simulink model "MdXX_RspOutComm"  (R2018b)
settings: Solver=FixedStepDiscrete  StartTime=0.0  StopTime=10.0  FixedStep=0.01  RelTol=1e-3
undefined symbols (not defined in the file or in its folder): KeSMSuRspStatHldTm_Val
libraries: RspLib x60
(part 2 of 2)

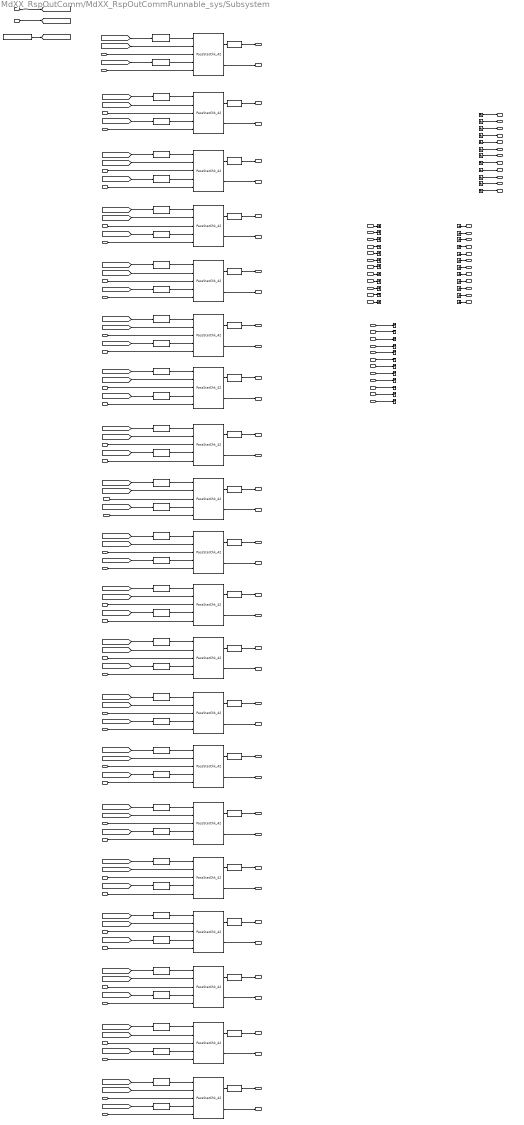
== system MdXX_RspOutComm/MdXX_RspOutCommRunnable_sys/Subsystem ==
  IsTargetPos32Bit_Val_read : Inport
  MdXX_Rsp_Md1_Rsp_read : Inport  Port=2
  MdXX_Rsp_Md10_Rsp_read : Inport  Port=3
  MdXX_Rsp_Md11_Rsp_read : Inport  Port=4
  MdXX_Rsp_Md12_Rsp_read : Inport  Port=5
  MdXX_Rsp_Md13_Rsp_read : Inport  Port=6
  MdXX_Rsp_Md14_Rsp_read : Inport  Port=7
  MdXX_Rsp_Md15_Rsp_read : Inport  Port=8
  MdXX_Rsp_Md16_Rsp_read : Inport  Port=9
  MdXX_Rsp_Md17_Rsp_read : Inport  Port=10
  MdXX_Rsp_Md18_Rsp_read : Inport  Port=11
  MdXX_Rsp_Md19_Rsp_read : Inport  Port=12
  MdXX_Rsp_Md2_Rsp_read : Inport  Port=13
  MdXX_Rsp_Md20_Rsp_read : Inport  Port=14
  MdXX_Rsp_Md21_Rsp_read : Inport  Port=15
  MdXX_Rsp_Md22_Rsp_read : Inport  Port=16
  MdXX_Rsp_Md23_Rsp_read : Inport  Port=17
  MdXX_Rsp_Md24_Rsp_read : Inport  Port=18
  MdXX_Rsp_Md25_Rsp_read : Inport  Port=19
  MdXX_Rsp_Md26_Rsp_read : Inport  Port=20
  MdXX_Rsp_Md27_Rsp_read : Inport  Port=21
  MdXX_Rsp_Md28_Rsp_read : Inport  Port=22
  MdXX_Rsp_Md29_Rsp_read : Inport  Port=23
  MdXX_Rsp_Md3_Rsp_read : Inport  Port=24
  MdXX_Rsp_Md30_Rsp_read : Inport  Port=25
  MdXX_Rsp_Md31_Rsp_read : Inport  Port=26
  MdXX_Rsp_Md32_Rsp_read : Inport  Port=27
  MdXX_Rsp_Md4_Rsp_read : Inport  Port=28
  MdXX_Rsp_Md5_Rsp_read : Inport  Port=29
  MdXX_Rsp_Md6_Rsp_read : Inport  Port=30
  MdXX_Rsp_Md7_Rsp_read : Inport  Port=31
  MdXX_Rsp_Md8_Rsp_read : Inport  Port=32
  MdXX_Rsp_Md9_Rsp_read : Inport  Port=33
  modestate32_Val_read : Inport  Port=34
  MdXX_SrcReqTp_Md1_SrcTp_read : Inport  Port=35
  MdXX_SrcReqTp_Md10_SrcTp_read : Inport  Port=36
  MdXX_SrcReqTp_Md11_SrcTp_read : Inport  Port=37
  MdXX_SrcReqTp_Md12_SrcTp_read : Inport  Port=38
  MdXX_SrcReqTp_Md13_SrcTp_read : Inport  Port=39
  MdXX_SrcReqTp_Md14_SrcTp_read : Inport  Port=40
  MdXX_SrcReqTp_Md15_SrcTp_read : Inport  Port=41
  MdXX_SrcReqTp_Md16_SrcTp_read : Inport  Port=42
  MdXX_SrcReqTp_Md17_SrcTp_read : Inport  Port=43
  MdXX_SrcReqTp_Md18_SrcTp_read : Inport  Port=44
  MdXX_SrcReqTp_Md19_SrcTp_read : Inport  Port=45
  MdXX_SrcReqTp_Md2_SrcTp_read : Inport  Port=46
  MdXX_SrcReqTp_Md20_SrcTp_read : Inport  Port=47
  MdXX_SrcReqTp_Md21_SrcTp_read : Inport  Port=48
  MdXX_SrcReqTp_Md22_SrcTp_read : Inport  Port=49
  MdXX_SrcReqTp_Md23_SrcTp_read : Inport  Port=50
  MdXX_SrcReqTp_Md24_SrcTp_read : Inport  Port=51
  MdXX_SrcReqTp_Md25_SrcTp_read : Inport  Port=52
  MdXX_SrcReqTp_Md26_SrcTp_read : Inport  Port=53
  MdXX_SrcReqTp_Md27_SrcTp_read : Inport  Port=54
  MdXX_SrcReqTp_Md28_SrcTp_read : Inport  Port=55
  MdXX_SrcReqTp_Md29_SrcTp_read : Inport  Port=56
  MdXX_SrcReqTp_Md3_SrcTp_read : Inport  Port=57
  MdXX_SrcReqTp_Md30_SrcTp_read : Inport  Port=58
  MdXX_SrcReqTp_Md31_SrcTp_read : Inport  Port=59
  MdXX_SrcReqTp_Md32_SrcTp_read : Inport  Port=60
  MdXX_SrcReqTp_Md4_SrcTp_read : Inport  Port=61
  MdXX_SrcReqTp_Md5_SrcTp_read : Inport  Port=62
  MdXX_SrcReqTp_Md6_SrcTp_read : Inport  Port=63
  MdXX_SrcReqTp_Md7_SrcTp_read : Inport  Port=64
  MdXX_SrcReqTp_Md8_SrcTp_read : Inport  Port=65
  MdXX_SrcReqTp_Md9_SrcTp_read : Inport  Port=66
  32BitSelector : RspLib/32BitSelector  BitNum=0
  32BitSelector1 : RspLib/32BitSelector  BitNum=0
  32BitSelector10 : RspLib/32BitSelector  BitNum=5
  32BitSelector11 : RspLib/32BitSelector  BitNum=5
  32BitSelector12 : RspLib/32BitSelector  BitNum=6
  32BitSelector13 : RspLib/32BitSelector  BitNum=6
  32BitSelector14 : RspLib/32BitSelector  BitNum=7
  32BitSelector15 : RspLib/32BitSelector  BitNum=7
  32BitSelector16 : RspLib/32BitSelector  BitNum=8
  32BitSelector17 : RspLib/32BitSelector  BitNum=8
  32BitSelector18 : RspLib/32BitSelector  BitNum=9
  32BitSelector19 : RspLib/32BitSelector  BitNum=9
  32BitSelector2 : RspLib/32BitSelector  BitNum=1
  32BitSelector20 : RspLib/32BitSelector  BitNum=10
  32BitSelector21 : RspLib/32BitSelector  BitNum=10
  32BitSelector22 : RspLib/32BitSelector  BitNum=11
  32BitSelector23 : RspLib/32BitSelector  BitNum=11
  32BitSelector24 : RspLib/32BitSelector  BitNum=12
  32BitSelector25 : RspLib/32BitSelector  BitNum=12
  32BitSelector26 : RspLib/32BitSelector  BitNum=13
  32BitSelector27 : RspLib/32BitSelector  BitNum=13
  32BitSelector28 : RspLib/32BitSelector  BitNum=14
  32BitSelector29 : RspLib/32BitSelector  BitNum=14
  32BitSelector3 : RspLib/32BitSelector  BitNum=1
  32BitSelector30 : RspLib/32BitSelector  BitNum=15
  32BitSelector31 : RspLib/32BitSelector  BitNum=15
  32BitSelector32 : RspLib/32BitSelector  BitNum=16
  32BitSelector33 : RspLib/32BitSelector  BitNum=16
  32BitSelector34 : RspLib/32BitSelector  BitNum=17
  32BitSelector35 : RspLib/32BitSelector  BitNum=17
  32BitSelector36 : RspLib/32BitSelector  BitNum=18
  32BitSelector37 : RspLib/32BitSelector  BitNum=18
  32BitSelector38 : RspLib/32BitSelector  BitNum=19
  32BitSelector39 : RspLib/32BitSelector  BitNum=19
  32BitSelector4 : RspLib/32BitSelector  BitNum=2
  32BitSelector5 : RspLib/32BitSelector  BitNum=2
  32BitSelector6 : RspLib/32BitSelector  BitNum=3
  32BitSelector7 : RspLib/32BitSelector  BitNum=3
  32BitSelector8 : RspLib/32BitSelector  BitNum=4
  32BitSelector9 : RspLib/32BitSelector  BitNum=4
  Data Type Conversion{1..20} (20 alike) : DataTypeConversion  OutDataTypeStr=uint8
  Ground_{1..12,14..22,24..26} (24 alike) : Ground
  Md10RspOutComm : RspLib/PassStatChk_42  SystemSampleTime=-1
  Md11RspOutComm : RspLib/PassStatChk_42  SystemSampleTime=-1
  Md12RspOutComm : RspLib/PassStatChk_42  SystemSampleTime=-1
  Md13RspOutComm : RspLib/PassStatChk_42  SystemSampleTime=-1
  Md14RspOutComm : RspLib/PassStatChk_42  SystemSampleTime=-1
  Md15RspOutComm : RspLib/PassStatChk_42  SystemSampleTime=-1
  Md16RspOutComm : RspLib/PassStatChk_42  SystemSampleTime=-1
  Md17RspOutComm : RspLib/PassStatChk_42  SystemSampleTime=-1
  Md18RspOutComm : RspLib/PassStatChk_42  SystemSampleTime=-1
  Md19RspOutComm : RspLib/PassStatChk_42  SystemSampleTime=-1
  Md1RspOutComm : RspLib/PassStatChk_42  SystemSampleTime=-1
  Md20RspOutComm : RspLib/PassStatChk_42  SystemSampleTime=-1
  Md2RspOutComm : RspLib/PassStatChk_42  SystemSampleTime=-1
  Md3RspOutComm : RspLib/PassStatChk_42  SystemSampleTime=-1
  Md4RspOutComm : RspLib/PassStatChk_42  SystemSampleTime=-1
  Md5RspOutComm : RspLib/PassStatChk_42  SystemSampleTime=-1
  Md6RspOutComm : RspLib/PassStatChk_42  SystemSampleTime=-1
  Md7RspOutComm : RspLib/PassStatChk_42  SystemSampleTime=-1
  Md8RspOutComm : RspLib/PassStatChk_42  SystemSampleTime=-1
  Md9RspOutComm : RspLib/PassStatChk_42  SystemSampleTime=-1
  PA_KeSMSuRspStatHldTm_Val : Constant  Value=KeSMSuRspStatHldTm_Val
  Terminator_{1..12,15..23,25..27} (24 alike) : Terminator
  MdXX_RspOutComm_Md1_Rsp_write : Outport
      settings: EnsureOutportIsVirtual=on
  MdXX_RspOutComm_Md10_Rsp_write : Outport  Port=2
      settings: EnsureOutportIsVirtual=on
  MdXX_RspOutComm_Md11_Rsp_write : Outport  Port=3
      settings: EnsureOutportIsVirtual=on
  MdXX_RspOutComm_Md12_Rsp_write : Outport  Port=4
      settings: EnsureOutportIsVirtual=on
  MdXX_RspOutComm_Md13_Rsp_write : Outport  Port=5
      settings: EnsureOutportIsVirtual=on
  MdXX_RspOutComm_Md14_Rsp_write : Outport  Port=6
      settings: EnsureOutportIsVirtual=on
  MdXX_RspOutComm_Md15_Rsp_write : Outport  Port=7
      settings: EnsureOutportIsVirtual=on
  MdXX_RspOutComm_Md16_Rsp_write : Outport  Port=8
      settings: EnsureOutportIsVirtual=on
  MdXX_RspOutComm_Md17_Rsp_write : Outport  Port=9
      settings: EnsureOutportIsVirtual=on
  MdXX_RspOutComm_Md18_Rsp_write : Outport  Port=10
      settings: EnsureOutportIsVirtual=on
  MdXX_RspOutComm_Md19_Rsp_write : Outport  Port=11
      settings: EnsureOutportIsVirtual=on
  MdXX_RspOutComm_Md2_Rsp_write : Outport  Port=12
      settings: EnsureOutportIsVirtual=on
  MdXX_RspOutComm_Md20_Rsp_write : Outport  Port=13
      settings: EnsureOutportIsVirtual=on
  MdXX_RspOutComm_Md21_Rsp_write : Outport  Port=14
      settings: EnsureOutportIsVirtual=on
  MdXX_RspOutComm_Md22_Rsp_write : Outport  Port=15
      settings: EnsureOutportIsVirtual=on
  MdXX_RspOutComm_Md23_Rsp_write : Outport  Port=16
      settings: EnsureOutportIsVirtual=on
  MdXX_RspOutComm_Md24_Rsp_write : Outport  Port=17
      settings: EnsureOutportIsVirtual=on
  MdXX_RspOutComm_Md25_Rsp_write : Outport  Port=18
      settings: EnsureOutportIsVirtual=on
  MdXX_RspOutComm_Md26_Rsp_write : Outport  Port=19
      settings: EnsureOutportIsVirtual=on
  MdXX_RspOutComm_Md27_Rsp_write : Outport  Port=20
      settings: EnsureOutportIsVirtual=on
  MdXX_RspOutComm_Md28_Rsp_write : Outport  Port=21
      settings: EnsureOutportIsVirtual=on
  MdXX_RspOutComm_Md29_Rsp_write : Outport  Port=22
      settings: EnsureOutportIsVirtual=on
  MdXX_RspOutComm_Md3_Rsp_write : Outport  Port=23
      settings: EnsureOutportIsVirtual=on
  MdXX_RspOutComm_Md30_Rsp_write : Outport  Port=24
      settings: EnsureOutportIsVirtual=on
  MdXX_RspOutComm_Md31_Rsp_write : Outport  Port=25
      settings: EnsureOutportIsVirtual=on
  MdXX_RspOutComm_Md32_Rsp_write : Outport  Port=26
      settings: EnsureOutportIsVirtual=on
  MdXX_RspOutComm_Md4_Rsp_write : Outport  Port=27
      settings: EnsureOutportIsVirtual=on
  MdXX_RspOutComm_Md5_Rsp_write : Outport  Port=28
      settings: EnsureOutportIsVirtual=on
  MdXX_RspOutComm_Md6_Rsp_write : Outport  Port=29
      settings: EnsureOutportIsVirtual=on
  MdXX_RspOutComm_Md7_Rsp_write : Outport  Port=30
      settings: EnsureOutportIsVirtual=on
  MdXX_RspOutComm_Md8_Rsp_write : Outport  Port=31
      settings: EnsureOutportIsVirtual=on
  MdXX_RspOutComm_Md9_Rsp_write : Outport  Port=32
      settings: EnsureOutportIsVirtual=on
  MdXX_SrcReqTpOutComm_Md1_SrcTp_write : Outport  Port=33
      settings: EnsureOutportIsVirtual=on
  MdXX_SrcReqTpOutComm_Md10_SrcTp_write : Outport  Port=34
      settings: EnsureOutportIsVirtual=on
  MdXX_SrcReqTpOutComm_Md11_SrcTp_write : Outport  Port=35
      settings: EnsureOutportIsVirtual=on
  MdXX_SrcReqTpOutComm_Md12_SrcTp_write : Outport  Port=36
      settings: EnsureOutportIsVirtual=on
  MdXX_SrcReqTpOutComm_Md13_SrcTp_write : Outport  Port=37
      settings: EnsureOutportIsVirtual=on
  MdXX_SrcReqTpOutComm_Md14_SrcTp_write : Outport  Port=38
      settings: EnsureOutportIsVirtual=on
  MdXX_SrcReqTpOutComm_Md15_SrcTp_write : Outport  Port=39
      settings: EnsureOutportIsVirtual=on
  MdXX_SrcReqTpOutComm_Md16_SrcTp_write : Outport  Port=40
      settings: EnsureOutportIsVirtual=on
  MdXX_SrcReqTpOutComm_Md17_SrcTp_write : Outport  Port=41
      settings: EnsureOutportIsVirtual=on
  MdXX_SrcReqTpOutComm_Md18_SrcTp_write : Outport  Port=42
      settings: EnsureOutportIsVirtual=on
  MdXX_SrcReqTpOutComm_Md19_SrcTp_write : Outport  Port=43
      settings: EnsureOutportIsVirtual=on
  MdXX_SrcReqTpOutComm_Md2_SrcTp_write : Outport  Port=44
      settings: EnsureOutportIsVirtual=on
  MdXX_SrcReqTpOutComm_Md20_SrcTp_write : Outport  Port=45
      settings: EnsureOutportIsVirtual=on
  MdXX_SrcReqTpOutComm_Md21_SrcTp_write : Outport  Port=46
      settings: EnsureOutportIsVirtual=on
  MdXX_SrcReqTpOutComm_Md22_SrcTp_write : Outport  Port=47
      settings: EnsureOutportIsVirtual=on
  MdXX_SrcReqTpOutComm_Md23_SrcTp_write : Outport  Port=48
      settings: EnsureOutportIsVirtual=on
  MdXX_SrcReqTpOutComm_Md24_SrcTp_write : Outport  Port=49
      settings: EnsureOutportIsVirtual=on
  MdXX_SrcReqTpOutComm_Md25_SrcTp_write : Outport  Port=50
      settings: EnsureOutportIsVirtual=on
  MdXX_SrcReqTpOutComm_Md26_SrcTp_write : Outport  Port=51
      settings: EnsureOutportIsVirtual=on
  MdXX_SrcReqTpOutComm_Md27_SrcTp_write : Outport  Port=52
      settings: EnsureOutportIsVirtual=on
  MdXX_SrcReqTpOutComm_Md28_SrcTp_write : Outport  Port=53
      settings: EnsureOutportIsVirtual=on
  MdXX_SrcReqTpOutComm_Md29_SrcTp_write : Outport  Port=54
      settings: EnsureOutportIsVirtual=on
  MdXX_SrcReqTpOutComm_Md3_SrcTp_write : Outport  Port=55
      settings: EnsureOutportIsVirtual=on
  MdXX_SrcReqTpOutComm_Md30_SrcTp_write : Outport  Port=56
      settings: EnsureOutportIsVirtual=on
  MdXX_SrcReqTpOutComm_Md31_SrcTp_write : Outport  Port=57
      settings: EnsureOutportIsVirtual=on
  MdXX_SrcReqTpOutComm_Md32_SrcTp_write : Outport  Port=58
      settings: EnsureOutportIsVirtual=on
  MdXX_SrcReqTpOutComm_Md4_SrcTp_write : Outport  Port=59
      settings: EnsureOutportIsVirtual=on
  MdXX_SrcReqTpOutComm_Md5_SrcTp_write : Outport  Port=60
      settings: EnsureOutportIsVirtual=on
  MdXX_SrcReqTpOutComm_Md6_SrcTp_write : Outport  Port=61
      settings: EnsureOutportIsVirtual=on
  MdXX_SrcReqTpOutComm_Md7_SrcTp_write : Outport  Port=62
      settings: EnsureOutportIsVirtual=on
  MdXX_SrcReqTpOutComm_Md8_SrcTp_write : Outport  Port=63
      settings: EnsureOutportIsVirtual=on
  MdXX_SrcReqTpOutComm_Md9_SrcTp_write : Outport  Port=64
      settings: EnsureOutportIsVirtual=on
  wires:
  MdXX_Rsp_Md5_Rsp_read/1 -> Md5RspOutComm/3
  Ground_19/1 -> MdXX_RspOutComm_Md26_Rsp_write/1
  Ground_16/1 -> MdXX_RspOutComm_Md23_Rsp_write/1
  MdXX_Rsp_Md26_Rsp_read/1 -> Terminator_20/1
  MdXX_Rsp_Md32_Rsp_read/1 -> Terminator_27/1
  Ground_22/1 -> MdXX_RspOutComm_Md29_Rsp_write/1
  MdXX_Rsp_Md23_Rsp_read/1 -> Terminator_17/1
  MdXX_Rsp_Md22_Rsp_read/1 -> Terminator_16/1
  Md16RspOutComm/1 -> Data Type Conversion16/1
  MdXX_Rsp_Md31_Rsp_read/1 -> Terminator_26/1
  Md15RspOutComm/1 -> Data Type Conversion15/1
  Md10RspOutComm/1 -> Data Type Conversion10/1
  MdXX_Rsp_Md2_Rsp_read/1 -> Md2RspOutComm/3
  Ground_18/1 -> MdXX_RspOutComm_Md25_Rsp_write/1
  Md13RspOutComm/1 -> Data Type Conversion13/1
  MdXX_Rsp_Md3_Rsp_read/1 -> Md3RspOutComm/3
  IsTargetPos32Bit_Val_read/1 -> [IsTargetPos32Bit]
  MdXX_Rsp_Md29_Rsp_read/1 -> Terminator_23/1
  Md18RspOutComm/1 -> Data Type Conversion18/1
  MdXX_Rsp_Md8_Rsp_read/1 -> Md8RspOutComm/3
  MdXX_Rsp_Md4_Rsp_read/1 -> Md4RspOutComm/3
  MdXX_Rsp_Md9_Rsp_read/1 -> Md9RspOutComm/3
  Ground_24/1 -> MdXX_RspOutComm_Md30_Rsp_write/1
  MdXX_Rsp_Md7_Rsp_read/1 -> Md7RspOutComm/3
  MdXX_Rsp_Md21_Rsp_read/1 -> Terminator_15/1
  Md12RspOutComm/1 -> Data Type Conversion12/1
  MdXX_Rsp_Md27_Rsp_read/1 -> Terminator_21/1
  MdXX_Rsp_Md28_Rsp_read/1 -> Terminator_22/1
  Ground_25/1 -> MdXX_RspOutComm_Md31_Rsp_write/1
  MdXX_Rsp_Md25_Rsp_read/1 -> Terminator_19/1
  MdXX_Rsp_Md24_Rsp_read/1 -> Terminator_18/1
  Md17RspOutComm/1 -> Data Type Conversion17/1
  MdXX_Rsp_Md6_Rsp_read/1 -> Md6RspOutComm/3
  Ground_21/1 -> MdXX_RspOutComm_Md28_Rsp_write/1
  modestate32_Val_read/1 -> [modestate32]
  Md19RspOutComm/1 -> Data Type Conversion19/1
  Ground_14/1 -> MdXX_RspOutComm_Md21_Rsp_write/1
  Ground_20/1 -> MdXX_RspOutComm_Md27_Rsp_write/1
  Md11RspOutComm/1 -> Data Type Conversion11/1
  Ground_15/1 -> MdXX_RspOutComm_Md22_Rsp_write/1
  Ground_17/1 -> MdXX_RspOutComm_Md24_Rsp_write/1
  Md14RspOutComm/1 -> Data Type Conversion14/1
  Md20RspOutComm/1 -> Data Type Conversion20/1
  Ground_26/1 -> MdXX_RspOutComm_Md32_Rsp_write/1
  MdXX_Rsp_Md30_Rsp_read/1 -> Terminator_25/1
  [IsTargetPos32Bit] -> 32BitSelector/1
  32BitSelector/1 -> Md1RspOutComm/4
  [modestate32] -> 32BitSelector1/1
  32BitSelector1/1 -> Md1RspOutComm/1
  PA_KeSMSuRspStatHldTm_Val/1 -> [KeSMSuRspStatHldTm_Val]
  [KeSMSuRspStatHldTm_Val] -> Md1RspOutComm/2
  MdXX_Rsp_Md1_Rsp_read/1 -> Md1RspOutComm/3
  Md1RspOutComm/1 -> Data Type Conversion1/1
  [KeSMSuRspStatHldTm_Val] -> Md2RspOutComm/2
  32BitSelector3/1 -> Md2RspOutComm/1
  [modestate32] -> 32BitSelector3/1
  32BitSelector2/1 -> Md2RspOutComm/4
  [IsTargetPos32Bit] -> 32BitSelector2/1
  [IsTargetPos32Bit] -> 32BitSelector4/1
  32BitSelector4/1 -> Md3RspOutComm/4
  [modestate32] -> 32BitSelector5/1
  32BitSelector5/1 -> Md3RspOutComm/1
  [KeSMSuRspStatHldTm_Val] -> Md3RspOutComm/2
  [KeSMSuRspStatHldTm_Val] -> Md4RspOutComm/2
  32BitSelector7/1 -> Md4RspOutComm/1
  [modestate32] -> 32BitSelector7/1
  32BitSelector6/1 -> Md4RspOutComm/4
  [IsTargetPos32Bit] -> 32BitSelector6/1
  [IsTargetPos32Bit] -> 32BitSelector8/1
  32BitSelector8/1 -> Md5RspOutComm/4
  [modestate32] -> 32BitSelector9/1
  32BitSelector9/1 -> Md5RspOutComm/1
  [KeSMSuRspStatHldTm_Val] -> Md5RspOutComm/2
  [KeSMSuRspStatHldTm_Val] -> Md6RspOutComm/2
  32BitSelector11/1 -> Md6RspOutComm/1
  [modestate32] -> 32BitSelector11/1
  32BitSelector10/1 -> Md6RspOutComm/4
  [IsTargetPos32Bit] -> 32BitSelector10/1
  [IsTargetPos32Bit] -> 32BitSelector12/1
  32BitSelector12/1 -> Md7RspOutComm/4
  [modestate32] -> 32BitSelector13/1
  32BitSelector13/1 -> Md7RspOutComm/1
  [KeSMSuRspStatHldTm_Val] -> Md7RspOutComm/2
  [KeSMSuRspStatHldTm_Val] -> Md8RspOutComm/2
  32BitSelector15/1 -> Md8RspOutComm/1
  [modestate32] -> 32BitSelector15/1
  32BitSelector14/1 -> Md8RspOutComm/4
  [IsTargetPos32Bit] -> 32BitSelector14/1
  [IsTargetPos32Bit] -> 32BitSelector16/1
  32BitSelector16/1 -> Md9RspOutComm/4
  [modestate32] -> 32BitSelector17/1
  32BitSelector17/1 -> Md9RspOutComm/1
  [KeSMSuRspStatHldTm_Val] -> Md9RspOutComm/2
  [KeSMSuRspStatHldTm_Val] -> Md10RspOutComm/2
  32BitSelector19/1 -> Md10RspOutComm/1
  [modestate32] -> 32BitSelector19/1
  32BitSelector18/1 -> Md10RspOutComm/4
  [IsTargetPos32Bit] -> 32BitSelector18/1
  Md2RspOutComm/1 -> Data Type Conversion2/1
  Md3RspOutComm/1 -> Data Type Conversion4/1
  Md4RspOutComm/1 -> Data Type Conversion3/1
  Md5RspOutComm/1 -> Data Type Conversion5/1
  Md6RspOutComm/1 -> Data Type Conversion6/1
  Md7RspOutComm/1 -> Data Type Conversion7/1
  Md8RspOutComm/1 -> Data Type Conversion8/1
  Md9RspOutComm/1 -> Data Type Conversion9/1
  [IsTargetPos32Bit] -> 32BitSelector20/1
  32BitSelector20/1 -> Md11RspOutComm/4
  [modestate32] -> 32BitSelector21/1
  32BitSelector21/1 -> Md11RspOutComm/1
  [KeSMSuRspStatHldTm_Val] -> Md11RspOutComm/2
  [KeSMSuRspStatHldTm_Val] -> Md12RspOutComm/2
  32BitSelector23/1 -> Md12RspOutComm/1
  [modestate32] -> 32BitSelector23/1
  32BitSelector22/1 -> Md12RspOutComm/4
  [IsTargetPos32Bit] -> 32BitSelector22/1
  [IsTargetPos32Bit] -> 32BitSelector24/1
  32BitSelector24/1 -> Md13RspOutComm/4
  [modestate32] -> 32BitSelector25/1
  32BitSelector25/1 -> Md13RspOutComm/1
  [KeSMSuRspStatHldTm_Val] -> Md13RspOutComm/2
  [KeSMSuRspStatHldTm_Val] -> Md14RspOutComm/2
  32BitSelector27/1 -> Md14RspOutComm/1
  [modestate32] -> 32BitSelector27/1
  32BitSelector26/1 -> Md14RspOutComm/4
  [IsTargetPos32Bit] -> 32BitSelector26/1
  [IsTargetPos32Bit] -> 32BitSelector28/1
  32BitSelector28/1 -> Md15RspOutComm/4
  [modestate32] -> 32BitSelector29/1
  32BitSelector29/1 -> Md15RspOutComm/1
  [KeSMSuRspStatHldTm_Val] -> Md15RspOutComm/2
  [KeSMSuRspStatHldTm_Val] -> Md16RspOutComm/2
  32BitSelector31/1 -> Md16RspOutComm/1
  [modestate32] -> 32BitSelector31/1
  32BitSelector30/1 -> Md16RspOutComm/4
  [IsTargetPos32Bit] -> 32BitSelector30/1
  [IsTargetPos32Bit] -> 32BitSelector32/1
  32BitSelector32/1 -> Md17RspOutComm/4
  [modestate32] -> 32BitSelector33/1
  32BitSelector33/1 -> Md17RspOutComm/1
  [KeSMSuRspStatHldTm_Val] -> Md17RspOutComm/2
  [KeSMSuRspStatHldTm_Val] -> Md18RspOutComm/2
  32BitSelector35/1 -> Md18RspOutComm/1
  [modestate32] -> 32BitSelector35/1
  32BitSelector34/1 -> Md18RspOutComm/4
  [IsTargetPos32Bit] -> 32BitSelector34/1
  [IsTargetPos32Bit] -> 32BitSelector36/1
  32BitSelector36/1 -> Md19RspOutComm/4
  [modestate32] -> 32BitSelector37/1
  32BitSelector37/1 -> Md19RspOutComm/1
  [KeSMSuRspStatHldTm_Val] -> Md19RspOutComm/2
  MdXX_Rsp_Md10_Rsp_read/1 -> Md10RspOutComm/3
  [KeSMSuRspStatHldTm_Val] -> Md20RspOutComm/2
  32BitSelector39/1 -> Md20RspOutComm/1
  [modestate32] -> 32BitSelector39/1
  32BitSelector38/1 -> Md20RspOutComm/4
  [IsTargetPos32Bit] -> 32BitSelector38/1
  MdXX_Rsp_Md11_Rsp_read/1 -> Md11RspOutComm/3
  MdXX_Rsp_Md12_Rsp_read/1 -> Md12RspOutComm/3
  MdXX_Rsp_Md13_Rsp_read/1 -> Md13RspOutComm/3
  MdXX_Rsp_Md14_Rsp_read/1 -> Md14RspOutComm/3
  MdXX_Rsp_Md15_Rsp_read/1 -> Md15RspOutComm/3
  MdXX_Rsp_Md16_Rsp_read/1 -> Md16RspOutComm/3
  MdXX_Rsp_Md17_Rsp_read/1 -> Md17RspOutComm/3
  MdXX_Rsp_Md18_Rsp_read/1 -> Md18RspOutComm/3
  MdXX_Rsp_Md19_Rsp_read/1 -> Md19RspOutComm/3
  MdXX_Rsp_Md20_Rsp_read/1 -> Md20RspOutComm/3
  Md1RspOutComm/2 -> MdXX_SrcReqTpOutComm_Md1_SrcTp_write/1
  Md4RspOutComm/2 -> MdXX_SrcReqTpOutComm_Md4_SrcTp_write/1
  Md5RspOutComm/2 -> MdXX_SrcReqTpOutComm_Md5_SrcTp_write/1
  Md6RspOutComm/2 -> MdXX_SrcReqTpOutComm_Md6_SrcTp_write/1
  Md7RspOutComm/2 -> MdXX_SrcReqTpOutComm_Md7_SrcTp_write/1
  Md8RspOutComm/2 -> MdXX_SrcReqTpOutComm_Md8_SrcTp_write/1
  Md9RspOutComm/2 -> MdXX_SrcReqTpOutComm_Md9_SrcTp_write/1
  Md10RspOutComm/2 -> MdXX_SrcReqTpOutComm_Md10_SrcTp_write/1
  Md11RspOutComm/2 -> MdXX_SrcReqTpOutComm_Md11_SrcTp_write/1
  Md12RspOutComm/2 -> MdXX_SrcReqTpOutComm_Md12_SrcTp_write/1
  Md13RspOutComm/2 -> MdXX_SrcReqTpOutComm_Md13_SrcTp_write/1
  Md14RspOutComm/2 -> MdXX_SrcReqTpOutComm_Md14_SrcTp_write/1
  Md15RspOutComm/2 -> MdXX_SrcReqTpOutComm_Md15_SrcTp_write/1
  Md16RspOutComm/2 -> MdXX_SrcReqTpOutComm_Md16_SrcTp_write/1
  Md17RspOutComm/2 -> MdXX_SrcReqTpOutComm_Md17_SrcTp_write/1
  Md18RspOutComm/2 -> MdXX_SrcReqTpOutComm_Md18_SrcTp_write/1
  Md19RspOutComm/2 -> MdXX_SrcReqTpOutComm_Md19_SrcTp_write/1
  Md20RspOutComm/2 -> MdXX_SrcReqTpOutComm_Md20_SrcTp_write/1
  Md2RspOutComm/2 -> MdXX_SrcReqTpOutComm_Md2_SrcTp_write/1
  Md3RspOutComm/2 -> MdXX_SrcReqTpOutComm_Md3_SrcTp_write/1
  Data Type Conversion3/1 -> MdXX_RspOutComm_Md4_Rsp_write/1
  Data Type Conversion4/1 -> MdXX_RspOutComm_Md3_Rsp_write/1
  Data Type Conversion2/1 -> MdXX_RspOutComm_Md2_Rsp_write/1
  Data Type Conversion1/1 -> MdXX_RspOutComm_Md1_Rsp_write/1
  Data Type Conversion5/1 -> MdXX_RspOutComm_Md5_Rsp_write/1
  Data Type Conversion6/1 -> MdXX_RspOutComm_Md6_Rsp_write/1
  Data Type Conversion7/1 -> MdXX_RspOutComm_Md7_Rsp_write/1
  Data Type Conversion8/1 -> MdXX_RspOutComm_Md8_Rsp_write/1
  Data Type Conversion9/1 -> MdXX_RspOutComm_Md9_Rsp_write/1
  Data Type Conversion10/1 -> MdXX_RspOutComm_Md10_Rsp_write/1
  Data Type Conversion11/1 -> MdXX_RspOutComm_Md11_Rsp_write/1
  Data Type Conversion12/1 -> MdXX_RspOutComm_Md12_Rsp_write/1
  Data Type Conversion13/1 -> MdXX_RspOutComm_Md13_Rsp_write/1
  Data Type Conversion14/1 -> MdXX_RspOutComm_Md14_Rsp_write/1
  Data Type Conversion15/1 -> MdXX_RspOutComm_Md15_Rsp_write/1
  Data Type Conversion16/1 -> MdXX_RspOutComm_Md16_Rsp_write/1
  Data Type Conversion17/1 -> MdXX_RspOutComm_Md17_Rsp_write/1
  Data Type Conversion18/1 -> MdXX_RspOutComm_Md18_Rsp_write/1
  Data Type Conversion19/1 -> MdXX_RspOutComm_Md19_Rsp_write/1
  Data Type Conversion20/1 -> MdXX_RspOutComm_Md20_Rsp_write/1
  Ground_1/1 -> MdXX_SrcReqTpOutComm_Md32_SrcTp_write/1
  Ground_2/1 -> MdXX_SrcReqTpOutComm_Md31_SrcTp_write/1
  Ground_3/1 -> MdXX_SrcReqTpOutComm_Md30_SrcTp_write/1
  Ground_4/1 -> MdXX_SrcReqTpOutComm_Md29_SrcTp_write/1
  Ground_5/1 -> MdXX_SrcReqTpOutComm_Md28_SrcTp_write/1
  Ground_6/1 -> MdXX_SrcReqTpOutComm_Md27_SrcTp_write/1
  Ground_7/1 -> MdXX_SrcReqTpOutComm_Md26_SrcTp_write/1
  Ground_8/1 -> MdXX_SrcReqTpOutComm_Md25_SrcTp_write/1
  Ground_9/1 -> MdXX_SrcReqTpOutComm_Md24_SrcTp_write/1
  Ground_10/1 -> MdXX_SrcReqTpOutComm_Md23_SrcTp_write/1
  Ground_11/1 -> MdXX_SrcReqTpOutComm_Md22_SrcTp_write/1
  Ground_12/1 -> MdXX_SrcReqTpOutComm_Md21_SrcTp_write/1
  MdXX_SrcReqTp_Md1_SrcTp_read/1 -> Md1RspOutComm/5
  MdXX_SrcReqTp_Md2_SrcTp_read/1 -> Md2RspOutComm/5
  MdXX_SrcReqTp_Md3_SrcTp_read/1 -> Md3RspOutComm/5
  MdXX_SrcReqTp_Md4_SrcTp_read/1 -> Md4RspOutComm/5
  MdXX_SrcReqTp_Md5_SrcTp_read/1 -> Md5RspOutComm/5
  MdXX_SrcReqTp_Md6_SrcTp_read/1 -> Md6RspOutComm/5
  MdXX_SrcReqTp_Md7_SrcTp_read/1 -> Md7RspOutComm/5
  MdXX_SrcReqTp_Md8_SrcTp_read/1 -> Md8RspOutComm/5
  MdXX_SrcReqTp_Md9_SrcTp_read/1 -> Md9RspOutComm/5
  MdXX_SrcReqTp_Md10_SrcTp_read/1 -> Md10RspOutComm/5
  MdXX_SrcReqTp_Md11_SrcTp_read/1 -> Md11RspOutComm/5
  MdXX_SrcReqTp_Md12_SrcTp_read/1 -> Md12RspOutComm/5
  MdXX_SrcReqTp_Md13_SrcTp_read/1 -> Md13RspOutComm/5
  MdXX_SrcReqTp_Md14_SrcTp_read/1 -> Md14RspOutComm/5
  MdXX_SrcReqTp_Md15_SrcTp_read/1 -> Md15RspOutComm/5
  MdXX_SrcReqTp_Md16_SrcTp_read/1 -> Md16RspOutComm/5
  MdXX_SrcReqTp_Md17_SrcTp_read/1 -> Md17RspOutComm/5
  MdXX_SrcReqTp_Md18_SrcTp_read/1 -> Md18RspOutComm/5
  MdXX_SrcReqTp_Md19_SrcTp_read/1 -> Md19RspOutComm/5
  MdXX_SrcReqTp_Md20_SrcTp_read/1 -> Md20RspOutComm/5
  MdXX_SrcReqTp_Md21_SrcTp_read/1 -> Terminator_1/1
  MdXX_SrcReqTp_Md22_SrcTp_read/1 -> Terminator_2/1
  MdXX_SrcReqTp_Md23_SrcTp_read/1 -> Terminator_3/1
  MdXX_SrcReqTp_Md24_SrcTp_read/1 -> Terminator_4/1
  MdXX_SrcReqTp_Md25_SrcTp_read/1 -> Terminator_5/1
  MdXX_SrcReqTp_Md26_SrcTp_read/1 -> Terminator_6/1
  MdXX_SrcReqTp_Md27_SrcTp_read/1 -> Terminator_7/1
  MdXX_SrcReqTp_Md28_SrcTp_read/1 -> Terminator_8/1
  MdXX_SrcReqTp_Md29_SrcTp_read/1 -> Terminator_9/1
  MdXX_SrcReqTp_Md30_SrcTp_read/1 -> Terminator_10/1
  MdXX_SrcReqTp_Md31_SrcTp_read/1 -> Terminator_11/1
  MdXX_SrcReqTp_Md32_SrcTp_read/1 -> Terminator_12/1
